simulink model "flex_sim"  (R2022a)
settings: Solver=ode45  StartTime=0.0  StopTime=3  MaxStep=0.01  RelTol=1e-4  AbsTol=1e-4
values from neighbouring files (symbols this model uses):
  B_b = 0.00056    [Example1.m]    (also in Example2.m = 0.003)
  B_m = 0.0048    [Example1.m]    (also in Example2.m = 0.003)
  B_s = 0.0004    [Example1.m]    (also in Example2.m = 0.003)
  J_c = J_m + J_f    (= 0.00344418071785)    [Example1.m]    (also in Example2.m)
  J_f = rho_flywheel*pi*D_flywheel^4*L_flywheel/32    (= 0.00340618071785)    [Example1.m]    (also in Example2.m)
  K = pi*G_shaft*D_shaft^4/(32*L_shaft)    (= 2.40616780706)    [Example1.m]    (also in Example2.m)
  K_m = 0.058    [Example1.m]    (also in Example2.m = 0.06)
  R_m = 1.4    [Example1.m]    (also in Example2.m = 0.9)
undefined symbols (not defined in the file or in its folder): freq
libraries: simulink x1
settings Model: Creator=jflaidla  LastModifiedBy=jflaidla
settings SolverCC: AutoScaleAbsTol=off  AlgebraicLoopSolver=TrustRegion
settings DataIOCC: SaveFormat=Array  SignalLoggingSaveFormat=ModelDataLogs  SaveOutput=off  SaveTime=off  ReturnWorkspaceOutputs=off
settings OptimizationCC: BooleanDataType=off  ExpressionDepthLimit=2147483647  InitFltsAndDblsToZero=on  LifeSpan=inf
settings DebuggingCC: SaveWithParameterizedLinksMsg=none  UnderspecifiedInitializationDetection=Classic  MergeDetectMultiDrivingBlocksExec=none  SignalResolutionControl=TryResolveAllWithWarning  MultiTaskDSMMsg=warning  MultiTaskCondExecSysMsg=none  FcnCallInpInsideContextMsg=warning  UnconnectedInputMsg=warning  UnconnectedOutputMsg=warning  UnconnectedLineMsg=warning  StateNameClashWarn=warning  SFUnexpectedBacktrackingDiag=warning  SFNoUnconditionalDefaultTransitionDiag=warning  SFExecutionAtInitializationDiag=none  SFMachineParentedDataDiag=warning  ArithmeticOperatorsInVariantConditions=warning
settings HardwareCC: ProdBitPerPointer=32  ProdBitPerSizeT=32  ProdBitPerPtrDiffT=32  ProdLargestAtomicFloat=None  ProdIntDivRoundTo=Undefined  ProdEndianess=Unspecified  ProdWordSize=32  ProdHWDeviceType=32-bit Generic  TargetUnknown=on
settings ModelReferenceCC: PropagateSignalLabelsOutOfModel=off
settings SFSimCC: SimUseLocalCustomCode=off  CustomCodeUndefinedFunction=UseInterfaceOnly
settings RTWCC: RTWUseLocalCustomCode=off
settings CodeAppCC: StateflowObjectComments=on
settings GRTTargetCC: TargetFcnLib=ansi_tfl_tmw.mat  TargetLangStandard=C89/C90 (ANSI)  CombineOutputUpdateFcns=off  GRTInterface=on
settings ConfigComp: CovMetricSettings=dw  CovSaveCumulativeToWorkspaceVar=on  CovSaveSingleToWorkspaceVar=on  CovExternalEMLEnable=off

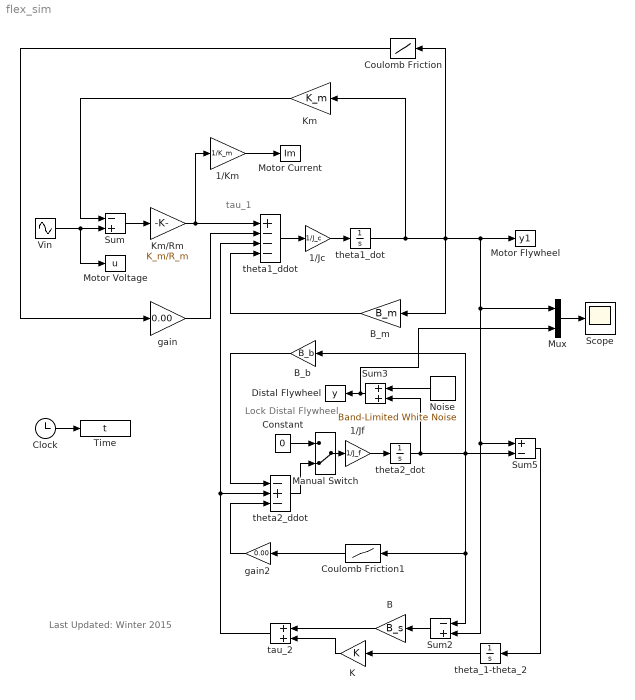
== system flex_sim ==
  note: tau_1
  note: Last Updated: Winter 2015
  note: Lock Distal
      | Flywheel
  1/Jc : Gain  Gain=1/J_c  SaturateOnIntegerOverflow=on  OutDataTypeStr=Inherit: Same as input  ParamDataTypeStr=Inherit: Same as input
  1/Jf : Gain  Gain=1/J_f  SaturateOnIntegerOverflow=on  OutDataTypeStr=Inherit: Same as input  ParamDataTypeStr=Inherit: Same as input
  1/Km : Gain  Gain=1/K_m  SaturateOnIntegerOverflow=on  OutDataTypeStr=Inherit: Same as input  ParamDataTypeStr=Inherit: Same as input
  B : Gain  Gain=B_s  SaturateOnIntegerOverflow=on  OutDataTypeStr=Inherit: Same as input  ParamDataTypeStr=Inherit: Same as input
  B_b : Gain  Gain=B_b  SaturateOnIntegerOverflow=on  OutDataTypeStr=Inherit: Same as input  ParamDataTypeStr=Inherit: Same as input
  B_m : Gain  Gain=B_m  SaturateOnIntegerOverflow=on  OutDataTypeStr=Inherit: Same as input  ParamDataTypeStr=Inherit: Same as input
  Clock : Clock
  Constant : Constant  Value=0
  Coulomb Friction : Lookup  InputValues=[-1,0,0,1]  Table=[-gain-ini -ini ini gain+ini]  mask(Coulombic Friction){ini=0, gain=1}
      mask prompts: ini "Offset discontinuity at zero:"
      mask help:
      | Coulombic Friction
      | y = sign(x) * (Gain * abs(x) + Offset)
      mask init:
      | x=max(ini,gain+ini);
      mask Help: This block has a discontinuity\nat zero and a linear gain afterward.\ny= sign(x)*(Gain*abs(x)+Offset)
      mask Display: plot([-1 0 0 1],[-gain-ini, -ini, ini, gain+ini],[-1 1],[0 0],[0 0],[-x,x])
  Coulomb Friction1 : Lookup  InputValues=[-1,0,0,1]  Table=[-gain-ini -ini ini gain+ini]  mask(Coulombic Friction){ini=0, gain=1}
      mask prompts: ini "Offset discontinuity at zero:"
      mask help:
      | Coulombic Friction
      | y = sign(x) * (Gain * abs(x) + Offset)
      mask init:
      | x=max(ini,gain+ini);
      mask Help: This block has a discontinuity\nat zero and a linear gain afterward.\ny= sign(x)*(Gain*abs(x)+Offset)
      mask Display: plot([-1 0 0 1],[-gain-ini, -ini, ini, gain+ini],[-1 1],[0 0],[0 0],[-x,x])
  Distal Flywheel : ToWorkspace  VariableName=y  SampleTime=0.01
      settings: MaxDataPoints=6001
  K : Gain  Gain=K  SaturateOnIntegerOverflow=on  OutDataTypeStr=Inherit: Same as input  ParamDataTypeStr=Inherit: Same as input
  Km : Gain  Gain=K_m  SaturateOnIntegerOverflow=on  OutDataTypeStr=Inherit: Same as input  ParamDataTypeStr=Inherit: Same as input
  Km/Rm : Gain  Gain=K_m/R_m  SaturateOnIntegerOverflow=on  OutDataTypeStr=Inherit: Same as input  ParamDataTypeStr=Inherit: Same as input
  Manual Switch : ManualSwitch  CurrentSetting=0
  Motor Current : ToWorkspace  VariableName=Im  SampleTime=0.01
      settings: MaxDataPoints=6001
  Motor Flywheel : ToWorkspace  VariableName=y1  SampleTime=0.01
      settings: MaxDataPoints=6001
  Motor Voltage : ToWorkspace  VariableName=u  SampleTime=0.01
      settings: MaxDataPoints=6001
  Mux : Mux  Inputs=2
  Noise : simulink/Sources/Band-Limited White Noise  Cov=[0.0]  Ts=0.01  seed=[23341]
  Scope : Scope
  Sum : Sum  Inputs=-+  InputSameDT=on  SaturateOnIntegerOverflow=on  OutDataTypeStr=Inherit: Same as first input
  Sum2 : Sum  Inputs=-+  InputSameDT=on  SaturateOnIntegerOverflow=on  OutDataTypeStr=Inherit: Same as first input
  Sum3 : Sum  InputSameDT=on  SaturateOnIntegerOverflow=on  SampleTime=0.01  OutDataTypeStr=Inherit: Same as first input
  Sum5 : Sum  Inputs=+-  InputSameDT=on  SaturateOnIntegerOverflow=on  OutDataTypeStr=Inherit: Same as first input
  Time : ToWorkspace  VariableName=t
      settings: MaxDataPoints=6001
  Vin : Sin  Frequency=freq  SampleTime=0
  gain : Gain  Gain=0.00  SaturateOnIntegerOverflow=on  OutDataTypeStr=Inherit: Same as input  ParamDataTypeStr=Inherit: Same as input
  gain2 : Gain  Gain=0.00  SaturateOnIntegerOverflow=on  OutDataTypeStr=Inherit: Same as input  ParamDataTypeStr=Inherit: Same as input
  tau_2 : Sum  InputSameDT=on  SaturateOnIntegerOverflow=on  OutDataTypeStr=Inherit: Same as first input
  theta1_ddot : Sum  Inputs=+---  InputSameDT=on  SaturateOnIntegerOverflow=on  OutDataTypeStr=Inherit: Same as first input
  theta1_dot : Integrator
  theta2_ddot : Sum  Inputs=-+-  InputSameDT=on  SaturateOnIntegerOverflow=on  OutDataTypeStr=Inherit: Same as first input
  theta2_dot : Integrator
  theta_1-theta_2 : Integrator
  wires:
  Sum/1 -> Km/Rm/1
  theta1_ddot/1 -> 1/Jc/1
  1/Jc/1 -> theta1_dot/1
  Vin/1 -> Sum/2, Motor Voltage/1
  Km/1 -> Sum/1
  Sum2/1 -> B/1
  B/1 -> tau_2/1
  K/1 -> tau_2/2
  theta2_dot/1 -> Sum2/1, Coulomb Friction1/1, Sum5/2, B_b/1, Sum3/2
  B_b/1 -> theta2_ddot/1
  tau_2/1 -> theta1_ddot/3, theta2_ddot/2
  theta2_ddot/1 -> Manual Switch/2
  1/Jf/1 -> theta2_dot/1
  Clock/1 -> Time/1
  Coulomb Friction/1 -> gain/1
  Coulomb Friction1/1 -> gain2/1
  gain2/1 -> theta2_ddot/3
  Sum5/1 -> theta_1-theta_2/1
  theta_1-theta_2/1 -> K/1
  Sum3/1 -> Mux/2, Distal Flywheel/1
  B_m/1 -> theta1_ddot/4
  gain/1 -> theta1_ddot/2
  Km/Rm/1 -> theta1_ddot/1, 1/Km/1
  1/Km/1 -> Motor Current/1
  Constant/1 -> Manual Switch/1
  Manual Switch/1 -> 1/Jf/1
  Noise/1 -> Sum3/1
  Mux/1 -> Scope/1
  theta1_dot/1 -> Km/1, Coulomb Friction/1, B_m/1, Motor Flywheel/1, Sum5/1, Sum2/2, Mux/1
